simulink model "analyze"  (R2014a)
settings: Solver=FixedStepDiscrete  StartTime=0.0  StopTime=1  FixedStep=0.02  RelTol=1e-3
InitFcn:
  | Veh_Par_wxt
values from neighbouring files (symbols this model uses):
  ag_thr = 0.4*g    (= 3.924)    [Veh_Par_wxt.m]
  B = 2.25    [Veh_Par_wxt.m]
  bra_pre_em = 12    [Veh_Par_wxt.m]
  bra_pre_gz2 = 12/3    (= 4)    [Veh_Par_wxt.m]
  bra_pre_gz34 = 12/3    (= 4)    [Veh_Par_wxt.m]
  bra_pre_yd = 12/2    (= 6)    [Veh_Par_wxt.m]
  brakepre_dem_data = [0 1 2 3 4 5 6 7 8 9 10 11 12]    [Veh_Par_wxt.m]
  brakeTrq_dem_data = [0 218.198 436.396 654.594 872.792 1090.99 1309.188 1527.386 1745.584 1963.782 2181.98 2400.178 2618.376]    [Veh_Par_wxt.m]
  bratrq_max = 4*2618.376    (= 10473.504)    [Veh_Par_wxt.m]
  eff_tran = 0.75    [Veh_Par_wxt.m]
  G = Mass*g    (= 36297)    [Veh_Par_wxt.m]
  kd1 = 1    [Veh_Par_wxt.m]
  kd2 = 1    [Veh_Par_wxt.m]
  kd3 = 1    [Veh_Par_wxt.m]
  ki1 = 1    [Veh_Par_wxt.m]
  ki2 = 1    [Veh_Par_wxt.m]
  ki3 = 1    [Veh_Par_wxt.m]
  kp1 = 1    [Veh_Par_wxt.m]
  kp2 = 1    [Veh_Par_wxt.m]
  kp3 = 1    [Veh_Par_wxt.m]
  L = 3.12    [Veh_Par_wxt.m]
  premax = 12    [Veh_Par_wxt.m]
  Radius = 0.20    (= 0.2)    [Veh_Par_wxt.m]
  s_opt_yi_add = 0.05    [Veh_Par_wxt.m]
  s_opt_zhuan_add = 0.05    [Veh_Par_wxt.m]
  spd_map_mot = [0 100 200 300 360 400 500 600 700 800 900]*tras_ratio    [Veh_Par_wxt.m]
  spdmax = 900*tras_ratio    (= 5580)    [Veh_Par_wxt.m]
  speed_thr_park = 5/3.6/Radius*30/pi    (= 66.3145596216)    [Veh_Par_wxt.m]
  tras_ratio = 6.2    [Veh_Par_wxt.m]
  trq_map_mot = [1200 1200 1200 1200 1200 1080 864 720 617 540 480]/tras_ratio    [Veh_Par_wxt.m]
  trqmax = 80    [Veh_Par_wxt.m]
  v_thr1_b = 5    [Veh_Par_wxt.m]
  v_thr2_b = 20    [Veh_Par_wxt.m]
  v_thr_park = 5    [Veh_Par_wxt.m]
undefined symbols (not defined in the file or in its folder): DiscIntNeverNeededParam
libraries: simulink x231, ec5744lib x19
(part 14 of 16)

== system analyze/MainControl/mode_control/forward/forward/Drive/驱动防滑控制TCS/转向TCS/右转 ==
  trq_dem_lf : Inport
  trq_dem_lr : Inport  Port=2
  trq_dem_rf : Inport  Port=3
  trq_dem_rr : Inport  Port=4
  bra_pre_l : Inport  Port=5
  bra_pre_r : Inport  Port=6
  s_act_lf : Inport  Port=7
  s_act_lr : Inport  Port=8
  s_act_rf : Inport  Port=9
  s_act_rr : Inport  Port=10
  brake_dem : Inport  Port=11
  s_opt_zhuan : Inport  Port=12
  Action Port : ActionPort  ActionType=case
  Constant{,1..3} (4 alike) : Constant  Value=s_opt_zhuan_add
  Constant4 : Constant  Value=0
  Constant5 : Constant  Value=0
  MATLAB Function : MATLAB Function  TreatAsAtomicUnit=on
  MATLAB Function1 : MATLAB Function  TreatAsAtomicUnit=on
  MATLAB Function2 : MATLAB Function  TreatAsAtomicUnit=on
  MATLAB Function3 : MATLAB Function  TreatAsAtomicUnit=on
  MATLAB Function4 : MATLAB Function  TreatAsAtomicUnit=on
  Memory{,1..3} (4 alike) : Memory  InheritSampleTime=on
  Multiport Switch : MultiPortSwitch  DataPortOrder=Zero-based contiguous  Inputs=4
  Mux{,1..3} (4 alike) : Mux  Inputs=6
  Switch Case : SwitchCase  CaseConditions={0,1,2,3}  ShowDefaultCase=off
  Terminator{,1..3} (4 alike) : Terminator
  前后轮均滑转 : Subsystem  TreatAsAtomicUnit=on
  前轮滑转 : Subsystem  TreatAsAtomicUnit=on
  后轮滑转 : Subsystem  TreatAsAtomicUnit=on
  无滑转 : Subsystem  TreatAsAtomicUnit=on
  forward_dem : Outport
  wires:
  Mux3/1 -> Multiport Switch/5
  [s_opt_zhuan] -> 前后轮均滑转/10(s_opt_zhuan)
  [s_act_lr] -> 前后轮均滑转/9(s_act_lr)
  [s_act_lf] -> 前后轮均滑转/8(s_act_lf)
  Switch Case/4 -> 前后轮均滑转/Action
  前后轮均滑转/6(bra_pre_r1) -> Mux3/6
  前后轮均滑转/5(bra_pre_l1) -> Mux3/5
  前后轮均滑转/4(mot_rr) -> Mux3/4
  前后轮均滑转/2(mot_lr) -> Mux3/2
  前后轮均滑转/3(mot_rf) -> Mux3/3
  前后轮均滑转/1(mot_lf) -> Mux3/1
  Switch Case/3 -> 后轮滑转/Action
  [s_opt_zhuan] -> 后轮滑转/9(s_opt_zhuan)
  [s_act_lr] -> 后轮滑转/8(s_act_lr)
  Mux2/1 -> Multiport Switch/4
  后轮滑转/6(bra_pre_r1) -> Mux2/6
  后轮滑转/5(bra_pre_l1) -> Mux2/5
  后轮滑转/4(mot_rr) -> Mux2/4
  后轮滑转/2(mot_lr) -> Mux2/2
  后轮滑转/3(mot_rf) -> Mux2/3
  后轮滑转/1(mot_lf) -> Mux2/1
  [s_opt_zhuan] -> 前轮滑转/9(s_opt_zhuan)
  [s_act_lf] -> 前轮滑转/8(s_act_lf)
  Mux1/1 -> Multiport Switch/3
  前轮滑转/4(mot_rr) -> Mux1/4
  前轮滑转/5(bra_pre_l1) -> Mux1/5
  前轮滑转/1(mot_lf) -> Mux1/1
  前轮滑转/2(mot_lr) -> Mux1/2
  前轮滑转/3(mot_rf) -> Mux1/3
  前轮滑转/6(bra_pre_r1) -> Mux1/6
  Switch Case/2 -> 前轮滑转/Action
  Multiport Switch/1 -> forward_dem/1
  Mux/1 -> Multiport Switch/2
  无滑转/6(bra_pre_r1) -> Mux/6
  无滑转/5(bra_pre_l1) -> Mux/5
  无滑转/3(mot_rf) -> Mux/3
  无滑转/4(mot_rr) -> Mux/4
  无滑转/2(mot_lr) -> Mux/2
  无滑转/1(mot_lf) -> Mux/1
  brake_dem/1 -> 前轮滑转/7(brake_dem), 后轮滑转/7(brake_dem), 前后轮均滑转/7(brake_dem), 无滑转/7(brake_dem)
  bra_pre_r/1 -> 前轮滑转/6(bra_pre_r), 后轮滑转/6(bra_pre_r), 前后轮均滑转/6(bra_pre_r), 无滑转/6(bra_pre_r)
  bra_pre_l/1 -> 前轮滑转/5(bra_pre_l), 后轮滑转/5(bra_pre_l), 前后轮均滑转/5(bra_pre_l), 无滑转/5(bra_pre_l)
  trq_dem_rr/1 -> 前轮滑转/4(trq_dem_rr), 后轮滑转/4(trq_dem_rr), 前后轮均滑转/4(trq_dem_rr), 无滑转/4(trq_dem_rr)
  trq_dem_rf/1 -> 前轮滑转/3(trq_dem_rf), 后轮滑转/3(trq_dem_rf), 前后轮均滑转/3(trq_dem_rf), 无滑转/3(trq_dem_rf)
  trq_dem_lr/1 -> 后轮滑转/2(trq_dem_lr), 前后轮均滑转/2(trq_dem_lr), 前轮滑转/2(trq_dem_lr), 无滑转/2(trq_dem_lr)
  trq_dem_lf/1 -> 前轮滑转/1(trq_dem_lf), 后轮滑转/1(trq_dem_lf), 前后轮均滑转/1(trq_dem_lf), 无滑转/1(trq_dem_lf)
  Switch Case/1 -> 无滑转/Action
  MATLAB Function4/1(y) -> Switch Case/1, Multiport Switch/1
  [flag_lr] -> MATLAB Function4/2(flag_lr)
  [flag_lf] -> MATLAB Function4/1(flag_lf)
  Constant3/1 -> MATLAB Function3/3(s_opt_zhuan_add)
  Memory3/1 -> MATLAB Function3/4(flag_rr_pre)
  MATLAB Function3/1(flag_rr) -> Terminator1/1, Memory3/1
  s_opt_zhuan/1 -> MATLAB Function/2(s_opt_zhuan), MATLAB Function1/2(s_opt_zhuan), MATLAB Function2/2(s_opt_zhuan), MATLAB Function3/2(s_opt_zhuan), [s_opt_zhuan]
  s_act_rr/1 -> MATLAB Function3/1(s_act_rr)
  Constant2/1 -> MATLAB Function2/3(s_opt_zhuan_add)
  Memory2/1 -> MATLAB Function2/4(flag_rf_pre)
  MATLAB Function2/1(flag_rf) -> Terminator/1, Memory2/1
  s_act_rf/1 -> MATLAB Function2/1(s_act_rf)
  Constant1/1 -> MATLAB Function1/3(s_opt_zhuan_add)
  Memory1/1 -> MATLAB Function1/4(flag_lr_pre)
  MATLAB Function1/1(flag_lr) -> Terminator3/1, Memory1/1
  s_act_lr/1 -> [s_act_lr], MATLAB Function1/1(s_act_lr)
  Constant/1 -> MATLAB Function/3(s_opt_zhuan_add)
  Memory/1 -> MATLAB Function/4(flag_lf_pre)
  MATLAB Function/1(flag_lf) -> Terminator2/1, Memory/1
  s_act_lf/1 -> [s_act_lf], MATLAB Function/1(s_act_lf)
  Constant4/1 -> [flag_lf]
  Constant5/1 -> [flag_lr]

== system analyze/MainControl/mode_control/forward/forward/Drive/驱动防滑控制TCS/转向TCS/左转 ==
  trq_dem_lf : Inport
  trq_dem_lr : Inport  Port=2
  trq_dem_rf : Inport  Port=3
  trq_dem_rr : Inport  Port=4
  bra_pre_l : Inport  Port=5
  bra_pre_r : Inport  Port=6
  s_act_lf : Inport  Port=7
  s_act_lr : Inport  Port=8
  s_act_rf : Inport  Port=9
  s_act_rr : Inport  Port=10
  brake_dem : Inport  Port=11
  s_opt_zhuan : Inport  Port=12
  Action Port : ActionPort  ActionType=case
  Constant{,1..3} (4 alike) : Constant  Value=s_opt_zhuan_add
  Constant4 : Constant  Value=0
  Constant5 : Constant  Value=0
  MATLAB Function : MATLAB Function  TreatAsAtomicUnit=on
  MATLAB Function1 : MATLAB Function  TreatAsAtomicUnit=on
  MATLAB Function2 : MATLAB Function  TreatAsAtomicUnit=on
  MATLAB Function3 : MATLAB Function  TreatAsAtomicUnit=on
  MATLAB Function4 : MATLAB Function  TreatAsAtomicUnit=on
  Memory{,1..3} (4 alike) : Memory  InheritSampleTime=on
  Multiport Switch : MultiPortSwitch  DataPortOrder=Zero-based contiguous  Inputs=4
  Mux{,1..3} (4 alike) : Mux  Inputs=6
  Switch Case : SwitchCase  CaseConditions={0,1,2,3}  ShowDefaultCase=off
  Terminator{,1..3} (4 alike) : Terminator
  前后轮均滑转 : Subsystem  TreatAsAtomicUnit=on
  前轮滑转 : Subsystem  TreatAsAtomicUnit=on
  后轮滑转 : Subsystem  TreatAsAtomicUnit=on
  无滑转 : Subsystem  TreatAsAtomicUnit=on
  forward_dem : Outport
  wires:
  s_act_lf/1 -> MATLAB Function/1(s_act_lf)
  MATLAB Function/1(flag_lf) -> Terminator/1, Memory/1
  Memory/1 -> MATLAB Function/4(flag_lf_pre)
  Constant/1 -> MATLAB Function/3(s_opt_zhuan_add)
  s_act_lr/1 -> MATLAB Function1/1(s_act_lr)
  MATLAB Function1/1(flag_lr) -> Terminator1/1, Memory1/1
  Memory1/1 -> MATLAB Function1/4(flag_lr_pre)
  Constant1/1 -> MATLAB Function1/3(s_opt_zhuan_add)
  s_act_rf/1 -> [s_act_rf], MATLAB Function2/1(s_act_rf)
  MATLAB Function2/1(flag_rf) -> Terminator2/1, Memory2/1
  Memory2/1 -> MATLAB Function2/4(flag_rf_pre)
  Constant2/1 -> MATLAB Function2/3(s_opt_zhuan_add)
  s_act_rr/1 -> [s_act_rr], MATLAB Function3/1(s_act_rr)
  s_opt_zhuan/1 -> [s_opt_zhuan], MATLAB Function3/2(s_opt_zhuan), MATLAB Function2/2(s_opt_zhuan), MATLAB Function1/2(s_opt_zhuan), MATLAB Function/2(s_opt_zhuan)
  MATLAB Function3/1(flag_rr) -> Terminator3/1, Memory3/1
  Memory3/1 -> MATLAB Function3/4(flag_rr_pre)
  Constant3/1 -> MATLAB Function3/3(s_opt_zhuan_add)
  [flag_rf] -> MATLAB Function4/1(flag_rf)
  [flag_rr] -> MATLAB Function4/2(flag_rr)
  MATLAB Function4/1(y) -> Multiport Switch/1, Switch Case/1
  Switch Case/1 -> 无滑转/Action
  trq_dem_lf/1 -> 无滑转/1(trq_dem_lf), 前后轮均滑转/1(trq_dem_lf), 后轮滑转/1(trq_dem_lf), 前轮滑转/1(trq_dem_lf)
  trq_dem_lr/1 -> 无滑转/2(trq_dem_lr), 前轮滑转/2(trq_dem_lr), 前后轮均滑转/2(trq_dem_lr), 后轮滑转/2(trq_dem_lr)
  trq_dem_rf/1 -> 无滑转/3(trq_dem_rf), 前后轮均滑转/3(trq_dem_rf), 后轮滑转/3(trq_dem_rf), 前轮滑转/3(trq_dem_rf)
  trq_dem_rr/1 -> 无滑转/4(trq_dem_rr), 前后轮均滑转/4(trq_dem_rr), 后轮滑转/4(trq_dem_rr), 前轮滑转/4(trq_dem_rr)
  bra_pre_l/1 -> 无滑转/5(bra_pre_l), 前后轮均滑转/5(bra_pre_l), 后轮滑转/5(bra_pre_l), 前轮滑转/5(bra_pre_l)
  bra_pre_r/1 -> 无滑转/6(bra_pre_r), 前后轮均滑转/6(bra_pre_r), 后轮滑转/6(bra_pre_r), 前轮滑转/6(bra_pre_r)
  brake_dem/1 -> 无滑转/7(brake_dem), 前后轮均滑转/7(brake_dem), 后轮滑转/7(brake_dem), 前轮滑转/7(brake_dem)
  无滑转/1(mot_lf) -> Mux/1
  无滑转/2(mot_lr) -> Mux/2
  无滑转/4(mot_rr) -> Mux/4
  无滑转/3(mot_rf) -> Mux/3
  无滑转/5(bra_pre_l1) -> Mux/5
  无滑转/6(bra_pre_r1) -> Mux/6
  Mux/1 -> Multiport Switch/2
  Multiport Switch/1 -> forward_dem/1
  Switch Case/2 -> 前轮滑转/Action
  前轮滑转/6(bra_pre_r1) -> Mux1/6
  前轮滑转/3(mot_rf) -> Mux1/3
  前轮滑转/2(mot_lr) -> Mux1/2
  前轮滑转/1(mot_lf) -> Mux1/1
  前轮滑转/5(bra_pre_l1) -> Mux1/5
  前轮滑转/4(mot_rr) -> Mux1/4
  Mux1/1 -> Multiport Switch/3
  [s_act_rf] -> 前轮滑转/8(s_act_rf)
  [s_opt_zhuan] -> 前轮滑转/9(s_opt_zhuan)
  后轮滑转/1(mot_lf) -> Mux2/1
  后轮滑转/3(mot_rf) -> Mux2/3
  后轮滑转/2(mot_lr) -> Mux2/2
  后轮滑转/4(mot_rr) -> Mux2/4
  后轮滑转/5(bra_pre_l1) -> Mux2/5
  后轮滑转/6(bra_pre_r1) -> Mux2/6
  Mux2/1 -> Multiport Switch/4
  [s_act_rr] -> 后轮滑转/8(s_act_rr)
  [s_opt_zhuan] -> 后轮滑转/9(s_opt_zhuan)
  Switch Case/3 -> 后轮滑转/Action
  前后轮均滑转/1(mot_lf) -> Mux3/1
  前后轮均滑转/3(mot_rf) -> Mux3/3
  前后轮均滑转/2(mot_lr) -> Mux3/2
  前后轮均滑转/4(mot_rr) -> Mux3/4
  前后轮均滑转/5(bra_pre_l1) -> Mux3/5
  前后轮均滑转/6(bra_pre_r1) -> Mux3/6
  Switch Case/4 -> 前后轮均滑转/Action
  [s_act_rf] -> 前后轮均滑转/8(s_act_rf)
  [s_act_rr] -> 前后轮均滑转/9(s_act_rr)
  [s_opt_zhuan] -> 前后轮均滑转/10(s_opt_zhuan)
  Mux3/1 -> Multiport Switch/5
  Constant4/1 -> [flag_rf]
  Constant5/1 -> [flag_rr]

== matlab function analyze/MainControl/mode_control/backward/backward/Drive/驱动防滑控制TCS/直行TCS/直行/HeartBeat ==
  data: life_pre input; life output
function life = fcn(life_pre)
%#codegen
life=life_pre+1;
if life>15
    life=0;
end
end

== matlab function analyze/MainControl/mode_control/backward/backward/Drive/驱动防滑控制TCS/直行TCS/直行/MATLAB Function4 ==
  data: trq_dem_lf input; trq_dem_lr input; trq_dem_rf input; trq_dem_rr input; bra_pre_l input; bra_pre_r input; brakepre_dem input; flag_lf input; flag_lr input; trq_out_lf output; flag_rf input; flag_rr input; trq_out_lr output; trq_out_rf output; trq_out_rr output; trq_pid_lf input; trq_pid_lr input; trq_pid_rf input; trq_pid_rr input; brapre_out_l output; brapre_out_r output; mode output
function [trq_out_lf,trq_out_lr,trq_out_rf,trq_out_rr,brapre_out_l,brapre_out_r,mode] = fcn(trq_dem_lf,trq_dem_lr,trq_dem_rf,trq_dem_rr,bra_pre_l,bra_pre_r,brakepre_dem,flag_lf,flag_lr,flag_rf,flag_rr,trq_pid_lf,trq_pid_lr,trq_pid_rf,trq_pid_rr)
%#codegen pid模块在外面做，里面进行十六种情况的判断，先看一下效果，不能再修改。
if flag_lf==0 && flag_lr==0 && flag_rf==0 && flag_rr==0 % 0电机滑转===============================================0电机滑转
    trq_out_lf=trq_dem_lf;
    trq_out_lr=trq_dem_lr;
    trq_out_rf=trq_dem_rf;
    trq_out_rr=trq_dem_rr;
    brapre_out_l=bra_pre_l+brakepre_dem;
    brapre_out_r=bra_pre_r+brakepre_dem;
    mode=1;
elseif flag_lf==1 && flag_lr==0 &&flag_rf==0 && flag_rr==0 %左前轮滑转===================================================1电机滑转
    trq_out_lf=trq_pid_lf;
    trq_out_lr=trq_dem_lr+(trq_dem_lf-trq_out_lf);
    trq_out_rf=trq_dem_rf;
    trq_out_rr=trq_dem_rr;
    brapre_out_l=bra_pre_l+brakepre_dem;
    brapre_out_r=bra_pre_r+brakepre_dem;
    mode=2;
elseif flag_lf==0 && flag_lr==1 &&flag_rf==0 && flag_rr==0 %左后轮滑转
    trq_out_lr=trq_pid_lr;
    trq_out_lf=trq_dem_lf+(trq_dem_lr-trq_out_lr);
    trq_out_rf=trq_dem_rf;
    trq_out_rr=trq_dem_rr;
    brapre_out_l=bra_pre_l+brakepre_dem;
    brapre_out_r=bra_pre_r+brakepre_dem;
    mode=3;
elseif flag_lf==0 && flag_lr==0 &&flag_rf==1 && flag_rr==0 %右前轮滑转
    trq_out_rf=trq_pid_rf;
    trq_out_rr=trq_dem_rr+(trq_dem_rf-trq_out_rf);
    trq_out_lf=trq_dem_lf;
    trq_out_lr=trq_dem_lr;
    brapre_out_l=bra_pre_l+brakepre_dem;
    brapre_out_r=bra_pre_r+brakepre_dem;
    mode=4;
elseif flag_lf==0 && flag_lr==0 &&flag_rf==0 && flag_rr==1 %右后轮滑转
    trq_out_rr=trq_pid_rr;
    trq_out_rf=trq_dem_rf+(trq_dem_rr-trq_out_rr);
    trq_out_lf=trq_dem_lf;
    trq_out_lr=trq_dem_lr;
    brapre_out_l=bra_pre_l+brakepre_dem;
    brapre_out_r=bra_pre_r+brakepre_dem;
    mode=5;
elseif flag_lf==1 && flag_lr==1 &&flag_rf==0 && flag_rr==0 %左侧两轮滑转=====================================================================2电机滑转
    trq_out_lf=trq_pid_lf;
    trq_out_lr=trq_pid_lr;
    trq_out_rf=trq_dem_rf-(trq_dem_lf+trq_dem_lr-trq_out_lf-trq_out_lr)/2;
    trq_out_rr=trq_dem_rr-(trq_dem_lf+trq_dem_lr-trq_out_lf-trq_out_lr)/2;
    brapre_out_l=bra_pre_l+brakepre_dem;
    brapre_out_r=bra_pre_r+brakepre_dem;
    mode=6;
elseif flag_lf==0 && flag_lr==0 &&flag_rf==1 && flag_rr==1 %右侧两轮滑转
    trq_out_rf=trq_pid_rf;
    trq_out_rr=trq_pid_rr;
    trq_out_lf=trq_dem_lf-(trq_dem_rf+trq_dem_rr-trq_out_rf-trq_out_rr)/2;
    trq_out_lr=trq_dem_lr-(trq_dem_rf+trq_dem_rr-trq_out_rf-trq_out_rr)/2;
    brapre_out_l=bra_pre_l+brakepre_dem;
    brapre_out_r=bra_pre_r+brakepre_dem;
    mode=7;
elseif flag_lf==1 && flag_lr==0 &&flag_rf==1 && flag_rr==0 %前轴滑转
    trq_out_lf=trq_pid_lf;
    trq_out_lr=trq_dem_lr+(trq_dem_lf-trq_out_lf);
    trq_out_rf=trq_pid_rf;
    trq_out_rr=trq_dem_rr+(trq_dem_rf-trq_out_rf);
    brapre_out_l=bra_pre_l+brakepre_dem;
    brapre_out_r=bra_pre_r+brakepre_dem;
    mode=8;
elseif flag_lf==0 && flag_lr==1 &&flag_rf==0 && flag_rr==1 %后轴滑转
    trq_out_lr=trq_pid_lr;
    trq_out_lf=trq_dem_lf+(trq_dem_lr-trq_out_lr);
    trq_out_rr=trq_pid_rr;
    trq_out_rf=trq_dem_rf+(trq_dem_rr-trq_out_rr);
    brapre_out_l=bra_pre_l+brakepre_dem;
    brapre_out_r=bra_pre_r+brakepre_dem;
    mode=9;
elseif flag_lf==1 && flag_lr==0 &&flag_rf==0 && flag_rr==1 %左前轮和右后轮滑转
    trq_out_lf=trq_pid_lf;
    trq_out_lr=trq_dem_lr+(trq_dem_lf-trq_out_lf);
    trq_out_rr=trq_pid_rr;
    trq_out_rf=trq_dem_rf+(trq_dem_rr-trq_out_rr);
    brapre_out_l=bra_pre_l+brakepre_dem;
    brapre_out_r=bra_pre_r+brakepre_dem;
    mode=10;
elseif flag_lf==0 && flag_lr==1 &&flag_rf==1 && flag_rr==0 %左后轮和右前轮滑转
    trq_out_lr=trq_pid_lr;
    trq_out_lf=trq_dem_lf+(trq_dem_lr-trq_out_lr);
    trq_out_rf=trq_pid_rf;
    trq_out_rr=trq_dem_rr+(trq_dem_rf-trq_out_rf);
    brapre_out_l=bra_pre_l+brakepre_dem;
    brapre_out_r=bra_pre_r+brakepre_dem;
    mode=11;
elseif flag_lf==1 && flag_lr==1 &&flag_rf==1 && flag_rr==0 %右后不滑转======================================================================3电机滑转
    trq_out_lf=trq_pid_lf;
    trq_out_lr=trq_pid_lr;
    trq_out_rf=trq_pid_rf;
    trq_out_rr=trq_dem_rr+(trq_dem_rf-trq_out_rf)-(trq_dem_lf+trq_dem_lr-trq_out_lf-trq_out_lr);
    brapre_out_l=bra_pre_l+brakepre_dem;
    brapre_out_r=bra_pre_r+brakepre_dem;
    mode=12;
elseif flag_lf==1 && flag_lr==1 &&flag_rf==0 && flag_rr==1 %右前不滑转
    trq_out_lf=trq_pid_lf;
    trq_out_lr=trq_pid_lr;
    trq_out_rr=trq_pid_rr;
    trq_out_rf=trq_dem_rf+(trq_dem_rr-trq_out_rr)-(trq_dem_lf+trq_dem_lr-trq_out_lf-trq_out_lr);
    brapre_out_l=bra_pre_l+brakepre_dem;
    brapre_out_r=bra_pre_r+brakepre_dem;
    mode=13;
elseif flag_lf==1 && flag_lr==0 &&flag_rf==1 && flag_rr==1 %左后不滑转
    trq_out_rf=trq_pid_rf;
    trq_out_rr=trq_pid_rr;
    trq_out_lf=trq_pid_lf;
    trq_out_lr=trq_dem_lr+(trq_dem_lf-trq_out_lf)-(trq_dem_rf+trq_dem_rr-trq_out_rf-trq_out_rr);
    brapre_out_l=bra_pre_l+brakepre_dem;
    brapre_out_r=bra_pre_r+brakepre_dem;
    mode=14;
elseif flag_lf==0 && flag_lr==1 &&flag_rf==1 && flag_rr==1 %左前不滑转
    trq_out_rf=trq_pid_rf;
    trq_out_rr=trq_pid_rr;
    trq_out_lr=trq_pid_lr;
    trq_out_lf=trq_dem_lf+(trq_dem_lr-trq_out_lr)-(trq_dem_rf+trq_dem_rr-trq_out_rf-trq_out_rr);
    brapre_out_l=bra_pre_l+brakepre_dem;
    brapre_out_r=bra_pre_r+brakepre_dem;
    mode=15;
else
    %     flag_lf==1 && flag_lr==1 &&flag_rf==1 && flag_rr==1 %4电机均滑转======================================================================4电机均滑转
    trqcha=(trq_pid_lf+trq_pid_lr)-(trq_pid_rf+trq_pid_rr);
    if trqcha>0
        trq_out_rf=trq_pid_rf;
        trq_out_rr=trq_pid_rr;
        trq_out_lf=trq_pid_lf-(trq_pid_lf/(trq_pid_lf+trq_pid_lr))*trqcha;
        trq_out_lr=trq_pid_lr-(trq_pid_lr/(trq_pid_lf+trq_pid_lr))*trqcha;
    else
        trq_out_lf=trq_pid_lf;
        trq_out_lr=trq_pid_lr;
        trq_out_rf=trq_pid_rf+(trq_pid_rf/(trq_pid_rf+trq_pid_rr))*trqcha;
        trq_out_rr=trq_pid_rr+(trq_pid_rr/(trq_pid_rf+trq_pid_rr))*trqcha;
    end
    brapre_out_l=bra_pre_l+brakepre_dem;
    brapre_out_r=bra_pre_r+brakepre_dem;
    mode=16;
end
trq_out_lf=max(0,trq_out_lf);
trq_out_lr=max(0,trq_out_lr);
trq_out_rf=max(0,trq_out_rf);
trq_out_rr=max(0,trq_out_rr);
brapre_out_l=brapre_out_l;
brapre_out_r=brapre_out_r;
end

== system analyze/MainControl/mode_control/backward/backward/Drive/驱动防滑控制TCS/直行TCS/直行/Subsystem ==
  s_opt_zhuan : Inport
  s_act_lf : Inport  Port=2
  s_act_lr : Inport  Port=3
  s_act_rf : Inport  Port=4
  s_act_rr : Inport  Port=5
  flag_lf : Inport  Port=6
  flag_lr : Inport  Port=7
  flag_rf : Inport  Port=8
  flag_rr : Inport  Port=9
  trq_dem_lf : Inport  Port=10
  trq_dem_lr : Inport  Port=11
  trq_dem_rf : Inport  Port=12
  trq_dem_rr : Inport  Port=13
  Add{1..2,5,7} (4 alike) : Sum  Inputs=+++
  Add{3..4,6,8} (4 alike) : Sum
  Difference{,1..3} (4 alike) : simulink/Discrete/Difference  ICPrevInput=0.0  InputProcessing=Inherited  OutMin=[]  OutMax=[]  OutDataType=fixdt(1, 16)  OutScaling=2^-10  DoSatur=off
  Discrete-Time Integrator{,1..3} (4 alike) : DiscreteIntegrator  SampleTime=-1  ICPrevOutput=DiscIntNeverNeededParam  ICPrevScaledInput=DiscIntNeverNeededParam
  Gain{1,4,7,10} (4 alike) : Gain  Gain=kp2
  Gain{2,5,8,11} (4 alike) : Gain  Gain=ki2
  Gain{3,6,9,12} (4 alike) : Gain  Gain=kd2
  Gain{13..16} (4 alike) : Gain  Gain=1/tras_ratio
  Sum{,1..3} (4 alike) : Sum  Inputs=|+-
  Switch{,1..3} (4 alike) : Switch  Criteria=u2 > Threshold  Threshold=0.5
  trq_pid_lf : Outport
  trq_pid_lr : Outport  Port=2
  trq_pid_rf : Outport  Port=3
  trq_pid_rr : Outport  Port=4
  wires:
  Difference2/1 -> Add5/3
  Discrete-Time Integrator2/1 -> Add5/2
  Difference3/1 -> Add7/3
  Discrete-Time Integrator3/1 -> Add7/2
  Difference1/1 -> Add1/3
  Discrete-Time Integrator1/1 -> Add1/2
  Difference/1 -> Add2/3
  Discrete-Time Integrator/1 -> Add2/2
  Add5/1 -> Gain16/1
  Sum2/1 -> Gain7/1, Gain9/1, Gain8/1
  Sum3/1 -> Gain10/1, Gain12/1, Gain11/1
  Add7/1 -> Gain15/1
  Gain6/1 -> Difference1/1
  Add1/1 -> Gain14/1
  Sum1/1 -> Gain4/1, Gain6/1, Gain5/1
  Sum/1 -> Gain1/1, Gain3/1, Gain2/1
  Add2/1 -> Gain13/1
  Switch3/1 -> trq_pid_rf/1
  flag_rf/1 -> Switch3/2
  [s_opt_zhuan] -> Sum3/1
  Gain10/1 -> Add7/1
  Gain11/1 -> Discrete-Time Integrator3/1
  Gain12/1 -> Difference3/1
  s_act_rf/1 -> Sum3/2
  trq_dem_rf/1 -> Add8/2, Switch3/3
  Add8/1 -> Switch3/1
  Switch2/1 -> trq_pid_rr/1
  flag_rr/1 -> Switch2/2
  [s_opt_zhuan] -> Sum2/1
  Gain7/1 -> Add5/1
  Gain8/1 -> Discrete-Time Integrator2/1
  Gain9/1 -> Difference2/1
  s_act_rr/1 -> Sum2/2
  trq_dem_rr/1 -> Add6/2, Switch2/3
  Add6/1 -> Switch2/1
  Switch1/1 -> trq_pid_lr/1
  flag_lr/1 -> Switch1/2
  [s_opt_zhuan] -> Sum1/1
  Gain4/1 -> Add1/1
  Gain5/1 -> Discrete-Time Integrator1/1
  s_act_lr/1 -> Sum1/2
  trq_dem_lr/1 -> Add4/2, Switch1/3
  Add4/1 -> Switch1/1
  Switch/1 -> trq_pid_lf/1
  flag_lf/1 -> Switch/2
  s_opt_zhuan/1 -> Sum/1, [s_opt_zhuan]
  Gain1/1 -> Add2/1
  Gain2/1 -> Discrete-Time Integrator/1
  Gain3/1 -> Difference/1
  s_act_lf/1 -> Sum/2
  trq_dem_lf/1 -> Add3/2, Switch/3
  Add3/1 -> Switch/1
  Gain13/1 -> Add3/1
  Gain14/1 -> Add4/1
  Gain15/1 -> Add8/1
  Gain16/1 -> Add6/1

== system analyze/MainControl/mode_control/backward/backward/Drive/驱动防滑控制TCS/直行TCS/直行/Subsystem1 ==
  brake_dem : Inport
  1-D Lookup Table : Lookup_n-D  NumberOfTableDimensions=1  BreakpointsForDimension1=brakeTrq_dem_data  Table=brakepre_dem_data  InternalRulePriority=Speed  RndMeth=Simplest  InputSameDT=on
  Constant : Constant  Value=bratrq_max
  Gain1 : Gain  Gain=1/2
  Gain2 : Gain  Gain=1/100
  Gain3 : Gain  Gain=1/2
  Product : Product
  brakepre_dem : Outport
  wires:
  brake_dem/1 -> Gain2/1
  Gain3/1 -> 1-D Lookup Table/1
  Gain2/1 -> Product/2
  Gain1/1 -> Gain3/1
  Product/1 -> Gain1/1
  Constant/1 -> Product/1
  1-D Lookup Table/1 -> brakepre_dem/1

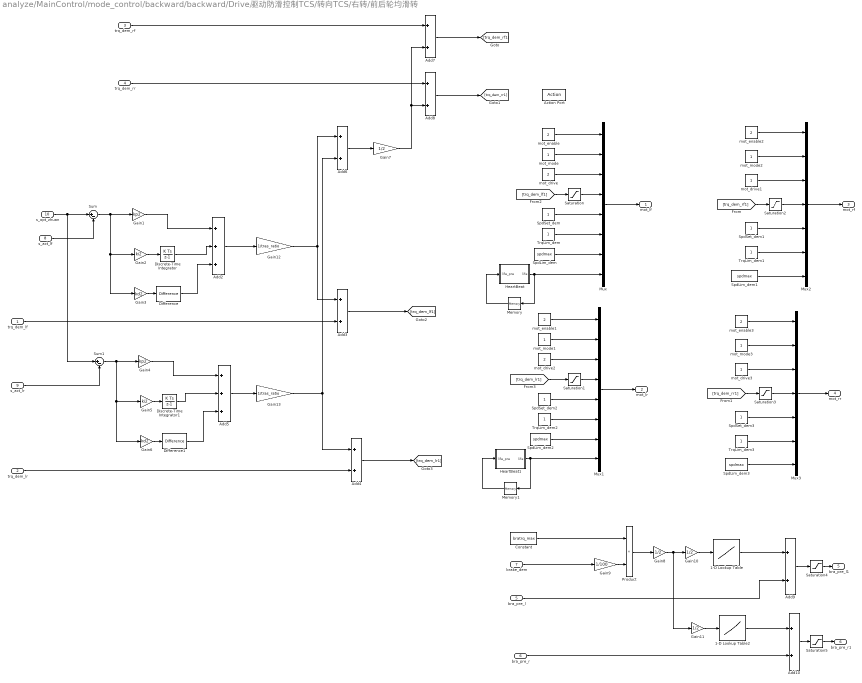
== system analyze/MainControl/mode_control/backward/backward/Drive/驱动防滑控制TCS/转向TCS/右转/前后轮均滑转 ==
  trq_dem_lf : Inport
  trq_dem_lr : Inport  Port=2
  trq_dem_rf : Inport  Port=3
  trq_dem_rr : Inport  Port=4
  bra_pre_l : Inport  Port=5
  bra_pre_r : Inport  Port=6
  brake_dem : Inport  Port=7
  s_act_lf : Inport  Port=8
  s_act_lr : Inport  Port=9
  s_opt_zhuan : Inport  Port=10
  Action Port : ActionPort  ActionType=case
  1-D Lookup Table : Lookup_n-D  NumberOfTableDimensions=1  BreakpointsForDimension1=brakeTrq_dem_data  Table=brakepre_dem_data  InternalRulePriority=Speed  RndMeth=Simplest  InputSameDT=on
  1-D Lookup Table2 : Lookup_n-D  NumberOfTableDimensions=1  BreakpointsForDimension1=brakeTrq_dem_data  Table=brakepre_dem_data  InternalRulePriority=Speed  RndMeth=Simplest  InputSameDT=on
  Add{3..4,6..10} (7 alike) : Sum
  Add2 : Sum  Inputs=+++
  Add5 : Sum  Inputs=+++
  Constant : Constant  Value=bratrq_max
  Difference : simulink/Discrete/Difference  ICPrevInput=0.0  InputProcessing=Inherited  OutMin=[]  OutMax=[]  OutDataType=fixdt(1, 16)  OutScaling=2^-10  DoSatur=off
  Difference1 : simulink/Discrete/Difference  ICPrevInput=0.0  InputProcessing=Inherited  OutMin=[]  OutMax=[]  OutDataType=fixdt(1, 16)  OutScaling=2^-10  DoSatur=off
  Discrete-Time Integrator : DiscreteIntegrator  SampleTime=-1  ICPrevOutput=DiscIntNeverNeededParam  ICPrevScaledInput=DiscIntNeverNeededParam
  Discrete-Time Integrator1 : DiscreteIntegrator  SampleTime=-1  ICPrevOutput=DiscIntNeverNeededParam  ICPrevScaledInput=DiscIntNeverNeededParam
  Gain1 : Gain  Gain=kp2
  Gain{7..8,10..11} (4 alike) : Gain  Gain=1/2
  Gain12 : Gain  Gain=1/tras_ratio
  Gain13 : Gain  Gain=1/tras_ratio
  Gain2 : Gain  Gain=ki2
  Gain3 : Gain  Gain=kd2
  Gain4 : Gain  Gain=kp2
  Gain5 : Gain  Gain=ki2
  Gain6 : Gain  Gain=kd2
  Gain9 : Gain  Gain=1/100
  HeartBeat : MATLAB Function  TreatAsAtomicUnit=on
  HeartBeat1 : MATLAB Function  TreatAsAtomicUnit=on
  Memory : Memory  InheritSampleTime=on
  Memory1 : Memory  InheritSampleTime=on
  Mux : Mux  Inputs=8
  Mux1 : Mux  Inputs=8
  Mux2 : Mux  Inputs=7
  Mux3 : Mux  Inputs=7
  Product : Product
  Saturation{,1..3} (4 alike) : Saturate  UpperLimit=trqmax  LowerLimit=-trqmax
  Saturation4 : Saturate  UpperLimit=premax  LowerLimit=0
  Saturation5 : Saturate  UpperLimit=premax  LowerLimit=0
  SpdLim_dem{,1..3} (4 alike) : Constant  Value=spdmax
  SpdSet_dem{,1..3} (4 alike) : Constant
  Sum : Sum  Inputs=|+-
  Sum1 : Sum  Inputs=|+-
  TrqLim_dem{,1..3} (4 alike) : Constant
  mot_drive : Constant  Value=2
  mot_drive1 : Constant
  mot_drive2 : Constant  Value=2
  mot_drive3 : Constant
  mot_enable{,1..3} (4 alike) : Constant  Value=2
  mot_mode{,1..3} (4 alike) : Constant
  mot_lf : Outport
  mot_lr : Outport  Port=2
  mot_rf : Outport  Port=3
  mot_rr : Outport  Port=4
  bra_pre_l1 : Outport  Port=5
  bra_pre_r1 : Outport  Port=6
  wires:
  Saturation5/1 -> bra_pre_r1/1
  Saturation4/1 -> bra_pre_l1/1
  Saturation3/1 -> Mux3/4
  Saturation2/1 -> Mux2/4
  Saturation1/1 -> Mux1/4
  Saturation/1 -> Mux/4
  Difference1/1 -> Add5/3
  Discrete-Time Integrator1/1 -> Add5/2
  Difference/1 -> Add2/3
  Discrete-Time Integrator/1 -> Add2/2
  Gain3/1 -> Difference/1
  brake_dem/1 -> Gain9/1
  Add10/1 -> Saturation5/1
  bra_pre_r/1 -> Add10/2
  1-D Lookup Table2/1 -> Add10/1
  Gain11/1 -> 1-D Lookup Table2/1
  Gain10/1 -> 1-D Lookup Table/1
  Gain9/1 -> Product/2
  Gain8/1 -> Gain10/1, Gain11/1
  Product/1 -> Gain8/1
  Constant/1 -> Product/1
  1-D Lookup Table/1 -> Add9/1
  Add9/1 -> Saturation4/1
  bra_pre_l/1 -> Add9/2
  SpdLim_dem3/1 -> Mux3/7
  TrqLim_dem3/1 -> Mux3/6
  Mux3/1 -> mot_rr/1
  SpdSet_dem3/1 -> Mux3/5
  mot_enable3/1 -> Mux3/1
  [trq_dem_rr1] -> Saturation3/1
  mot_mode3/1 -> Mux3/2
  mot_drive3/1 -> Mux3/3
  SpdLim_dem2/1 -> Mux1/7
  Memory1/1 -> HeartBeat1/1(life_pre)
  HeartBeat1/1(life) -> Memory1/1, Mux1/8
  TrqLim_dem2/1 -> Mux1/6
  Mux1/1 -> mot_lr/1
  SpdSet_dem2/1 -> Mux1/5
  mot_enable1/1 -> Mux1/1
  [trq_dem_lr1] -> Saturation1/1
  mot_mode1/1 -> Mux1/2
  mot_drive2/1 -> Mux1/3
  SpdLim_dem1/1 -> Mux2/7
  TrqLim_dem1/1 -> Mux2/6
  Mux2/1 -> mot_rf/1
  SpdSet_dem1/1 -> Mux2/5
  mot_enable2/1 -> Mux2/1
  [trq_dem_rf1] -> Saturation2/1
  mot_mode2/1 -> Mux2/2
  mot_drive1/1 -> Mux2/3
  SpdLim_dem/1 -> Mux/7
  Memory/1 -> HeartBeat/1(life_pre)
  HeartBeat/1(life) -> Memory/1, Mux/8
  TrqLim_dem/1 -> Mux/6
  Mux/1 -> mot_lf/1
  SpdSet_dem/1 -> Mux/5
  mot_enable/1 -> Mux/1
  [trq_dem_lf1] -> Saturation/1
  mot_mode/1 -> Mux/2
  mot_drive/1 -> Mux/3
  s_opt_zhuan/1 -> Sum1/1, Sum/1
  Sum/1 -> Gain2/1, Gain3/1, Gain1/1
  Gain1/1 -> Add2/1
  Gain2/1 -> Discrete-Time Integrator/1
  s_act_lf/1 -> Sum/2
  Add2/1 -> Gain12/1
  trq_dem_lf/1 -> Add3/2
  Add3/1 -> [trq_dem_lf1]
  Add4/1 -> [trq_dem_lr1]
  Sum1/1 -> Gain5/1, Gain6/1, Gain4/1
  Gain4/1 -> Add5/1
  Gain5/1 -> Discrete-Time Integrator1/1
  Gain6/1 -> Difference1/1
  s_act_lr/1 -> Sum1/2
  Add5/1 -> Gain13/1
  trq_dem_lr/1 -> Add4/2
  Add6/1 -> Gain7/1
  trq_dem_rf/1 -> Add7/1
  Gain7/1 -> Add8/2, Add7/2
  Add7/1 -> [trq_dem_rf1]
  trq_dem_rr/1 -> Add8/1
  Add8/1 -> [trq_dem_rr1]
  Gain12/1 -> Add3/1, Add6/1
  Gain13/1 -> Add4/1, Add6/2

== system analyze/MainControl/mode_control/backward/backward/Drive/驱动防滑控制TCS/转向TCS/右转/前轮滑转 ==
  trq_dem_lf : Inport
  trq_dem_lr : Inport  Port=2
  trq_dem_rf : Inport  Port=3
  trq_dem_rr : Inport  Port=4
  bra_pre_l : Inport  Port=5
  bra_pre_r : Inport  Port=6
  brake_dem : Inport  Port=7
  s_act_lf : Inport  Port=8
  s_opt_zhuan : Inport  Port=9
  Action Port : ActionPort  ActionType=case
  1-D Lookup Table : Lookup_n-D  NumberOfTableDimensions=1  BreakpointsForDimension1=brakeTrq_dem_data  Table=brakepre_dem_data  InternalRulePriority=Speed  RndMeth=Simplest  InputSameDT=on
  1-D Lookup Table2 : Lookup_n-D  NumberOfTableDimensions=1  BreakpointsForDimension1=brakeTrq_dem_data  Table=brakepre_dem_data  InternalRulePriority=Speed  RndMeth=Simplest  InputSameDT=on
  Add2 : Sum  Inputs=+++
  Add{3..6} (4 alike) : Sum
  Constant : Constant  Value=bratrq_max
  Difference : simulink/Discrete/Difference  ICPrevInput=0.0  InputProcessing=Inherited  OutMin=[]  OutMax=[]  OutDataType=fixdt(1, 16)  OutScaling=2^-10  DoSatur=off
  Discrete-Time Integrator : DiscreteIntegrator  SampleTime=-1  ICPrevOutput=DiscIntNeverNeededParam  ICPrevScaledInput=DiscIntNeverNeededParam
  Gain1 : Gain  Gain=kp2
  Gain2 : Gain  Gain=ki2
  Gain3 : Gain  Gain=kd2
  Gain4 : Gain  Gain=-1
  Gain5 : Gain  Gain=1/2
  Gain6 : Gain  Gain=1/100
  Gain7 : Gain  Gain=1/2
  Gain8 : Gain  Gain=1/2
  Gain9 : Gain  Gain=1/tras_ratio
  HeartBeat : MATLAB Function  TreatAsAtomicUnit=on
  HeartBeat1 : MATLAB Function  TreatAsAtomicUnit=on
  Memory : Memory  InheritSampleTime=on
  Memory1 : Memory  InheritSampleTime=on
  Mux : Mux  Inputs=8
  Mux1 : Mux  Inputs=8
  Mux2 : Mux  Inputs=7
  Mux3 : Mux  Inputs=7
  Product : Product
  Saturation{,1..3} (4 alike) : Saturate  UpperLimit=trqmax  LowerLimit=-trqmax
  Saturation4 : Saturate  UpperLimit=premax  LowerLimit=0
  Saturation5 : Saturate  UpperLimit=premax  LowerLimit=0
  SpdLim_dem{,1..3} (4 alike) : Constant  Value=spdmax
  SpdSet_dem{,1..3} (4 alike) : Constant
  Sum : Sum  Inputs=|+-
  TrqLim_dem{,1..3} (4 alike) : Constant
  mot_drive : Constant  Value=2
  mot_drive1 : Constant
  mot_drive2 : Constant  Value=2
  mot_drive3 : Constant
  mot_enable{,1..3} (4 alike) : Constant  Value=2
  mot_mode{,1..3} (4 alike) : Constant
  mot_lf : Outport
  mot_lr : Outport  Port=2
  mot_rf : Outport  Port=3
  mot_rr : Outport  Port=4
  bra_pre_l1 : Outport  Port=5
  bra_pre_r1 : Outport  Port=6
  wires:
  Saturation5/1 -> bra_pre_r1/1
  Saturation4/1 -> bra_pre_l1/1
  Saturation3/1 -> Mux3/4
  Saturation2/1 -> Mux2/4
  Saturation1/1 -> Mux1/4
  Saturation/1 -> Mux/4
  Difference/1 -> Add2/3
  Discrete-Time Integrator/1 -> Add2/2
  brake_dem/1 -> Gain6/1
  Add6/1 -> Saturation5/1
  bra_pre_r/1 -> Add6/2
  1-D Lookup Table2/1 -> Add6/1
  Gain8/1 -> 1-D Lookup Table2/1
  Gain7/1 -> 1-D Lookup Table/1
  Gain6/1 -> Product/2
  Gain5/1 -> Gain7/1, Gain8/1
  Product/1 -> Gain5/1
  Constant/1 -> Product/1
  1-D Lookup Table/1 -> Add5/1
  Add5/1 -> Saturation4/1
  bra_pre_l/1 -> Add5/2
  SpdLim_dem3/1 -> Mux3/7
  TrqLim_dem3/1 -> Mux3/6
  Mux3/1 -> mot_rr/1
  SpdSet_dem3/1 -> Mux3/5
  mot_enable3/1 -> Mux3/1
  trq_dem_rr/1 -> Saturation3/1
  mot_mode3/1 -> Mux3/2
  mot_drive3/1 -> Mux3/3
  SpdLim_dem2/1 -> Mux1/7
  Memory1/1 -> HeartBeat1/1(life_pre)
  HeartBeat1/1(life) -> Memory1/1, Mux1/8
  TrqLim_dem2/1 -> Mux1/6
  Mux1/1 -> mot_lr/1
  SpdSet_dem2/1 -> Mux1/5
  mot_enable1/1 -> Mux1/1
  [trq_dem_lr1] -> Saturation1/1
  mot_mode1/1 -> Mux1/2
  mot_drive2/1 -> Mux1/3
  SpdLim_dem1/1 -> Mux2/7
  TrqLim_dem1/1 -> Mux2/6
  Mux2/1 -> mot_rf/1
  SpdSet_dem1/1 -> Mux2/5
  mot_enable2/1 -> Mux2/1
  trq_dem_rf/1 -> Saturation2/1
  mot_mode2/1 -> Mux2/2
  mot_drive1/1 -> Mux2/3
  SpdLim_dem/1 -> Mux/7
  Memory/1 -> HeartBeat/1(life_pre)
  HeartBeat/1(life) -> Memory/1, Mux/8
  TrqLim_dem/1 -> Mux/6
  Mux/1 -> mot_lf/1
  SpdSet_dem/1 -> Mux/5
  mot_enable/1 -> Mux/1
  [trq_dem_lf1] -> Saturation/1
  mot_mode/1 -> Mux/2
  mot_drive/1 -> Mux/3
  s_opt_zhuan/1 -> Sum/1
  Sum/1 -> Gain2/1, Gain3/1, Gain1/1
  Gain1/1 -> Add2/1
  Gain2/1 -> Discrete-Time Integrator/1
  Gain3/1 -> Difference/1
  s_act_lf/1 -> Sum/2
  Add2/1 -> Gain9/1
  trq_dem_lf/1 -> Add3/2
  Add3/1 -> [trq_dem_lf1]
  Gain4/1 -> Add4/1
  trq_dem_lr/1 -> Add4/2
  Add4/1 -> [trq_dem_lr1]
  Gain9/1 -> Gain4/1, Add3/1

== system analyze/MainControl/mode_control/backward/backward/Drive/驱动防滑控制TCS/转向TCS/右转/后轮滑转 ==
  trq_dem_lf : Inport
  trq_dem_lr : Inport  Port=2
  trq_dem_rf : Inport  Port=3
  trq_dem_rr : Inport  Port=4
  bra_pre_l : Inport  Port=5
  bra_pre_r : Inport  Port=6
  brake_dem : Inport  Port=7
  s_act_lr : Inport  Port=8
  s_opt_zhuan : Inport  Port=9
  Action Port : ActionPort  ActionType=case
  1-D Lookup Table : Lookup_n-D  NumberOfTableDimensions=1  BreakpointsForDimension1=brakeTrq_dem_data  Table=brakepre_dem_data  InternalRulePriority=Speed  RndMeth=Simplest  InputSameDT=on
  1-D Lookup Table2 : Lookup_n-D  NumberOfTableDimensions=1  BreakpointsForDimension1=brakeTrq_dem_data  Table=brakepre_dem_data  InternalRulePriority=Speed  RndMeth=Simplest  InputSameDT=on
  Add2 : Sum  Inputs=+++
  Add{3..6} (4 alike) : Sum
  Constant : Constant  Value=bratrq_max
  Difference : simulink/Discrete/Difference  ICPrevInput=0.0  InputProcessing=Inherited  OutMin=[]  OutMax=[]  OutDataType=fixdt(1, 16)  OutScaling=2^-10  DoSatur=off
  Discrete-Time Integrator : DiscreteIntegrator  SampleTime=-1  ICPrevOutput=DiscIntNeverNeededParam  ICPrevScaledInput=DiscIntNeverNeededParam
  Gain1 : Gain  Gain=kp2
  Gain2 : Gain  Gain=ki2
  Gain3 : Gain  Gain=kd2
  Gain4 : Gain  Gain=-1
  Gain5 : Gain  Gain=1/2
  Gain6 : Gain  Gain=1/100
  Gain7 : Gain  Gain=1/2
  Gain8 : Gain  Gain=1/2
  Gain9 : Gain  Gain=1/tras_ratio
  HeartBeat : MATLAB Function  TreatAsAtomicUnit=on
  HeartBeat1 : MATLAB Function  TreatAsAtomicUnit=on
  Memory : Memory  InheritSampleTime=on
  Memory1 : Memory  InheritSampleTime=on
  Mux : Mux  Inputs=8
  Mux1 : Mux  Inputs=8
  Mux2 : Mux  Inputs=7
  Mux3 : Mux  Inputs=7
  Product : Product
  Saturation{,1..3} (4 alike) : Saturate  UpperLimit=trqmax  LowerLimit=-trqmax
  Saturation4 : Saturate  UpperLimit=premax  LowerLimit=0
  Saturation5 : Saturate  UpperLimit=premax  LowerLimit=0
  SpdLim_dem{,1..3} (4 alike) : Constant  Value=spdmax
  SpdSet_dem{,1..3} (4 alike) : Constant
  Sum : Sum  Inputs=|+-
  TrqLim_dem{,1..3} (4 alike) : Constant
  mot_drive : Constant  Value=2
  mot_drive1 : Constant
  mot_drive2 : Constant  Value=2
  mot_drive3 : Constant
  mot_enable{,1..3} (4 alike) : Constant  Value=2
  mot_mode{,1..3} (4 alike) : Constant
  mot_lf : Outport
  mot_lr : Outport  Port=2
  mot_rf : Outport  Port=3
  mot_rr : Outport  Port=4
  bra_pre_l1 : Outport  Port=5
  bra_pre_r1 : Outport  Port=6
  wires:
  Saturation5/1 -> bra_pre_r1/1
  Saturation4/1 -> bra_pre_l1/1
  Saturation3/1 -> Mux3/4
  Saturation2/1 -> Mux2/4
  Saturation1/1 -> Mux1/4
  Saturation/1 -> Mux/4
  Difference/1 -> Add2/3
  Discrete-Time Integrator/1 -> Add2/2
  brake_dem/1 -> Gain6/1
  Add6/1 -> Saturation5/1
  bra_pre_r/1 -> Add6/2
  1-D Lookup Table2/1 -> Add6/1
  Gain8/1 -> 1-D Lookup Table2/1
  Gain7/1 -> 1-D Lookup Table/1
  Gain6/1 -> Product/2
  Gain5/1 -> Gain7/1, Gain8/1
  Product/1 -> Gain5/1
  Constant/1 -> Product/1
  1-D Lookup Table/1 -> Add5/1
  Add5/1 -> Saturation4/1
  bra_pre_l/1 -> Add5/2
  Add4/1 -> [trq_dem_lf1]
  trq_dem_lf/1 -> Add4/2
  Gain4/1 -> Add4/1
  Add3/1 -> [trq_dem_lr1]
  trq_dem_lr/1 -> Add3/2
  Add2/1 -> Gain9/1
  s_act_lr/1 -> Sum/2
  Gain3/1 -> Difference/1
  Gain2/1 -> Discrete-Time Integrator/1
  Gain1/1 -> Add2/1
  Sum/1 -> Gain1/1, Gain3/1, Gain2/1
  s_opt_zhuan/1 -> Sum/1
  mot_drive/1 -> Mux/3
  mot_mode/1 -> Mux/2
  [trq_dem_lf1] -> Saturation/1
  mot_enable/1 -> Mux/1
  SpdSet_dem/1 -> Mux/5
  Mux/1 -> mot_lf/1
  TrqLim_dem/1 -> Mux/6
  HeartBeat/1(life) -> Mux/8, Memory/1
  Memory/1 -> HeartBeat/1(life_pre)
  SpdLim_dem/1 -> Mux/7
  mot_drive1/1 -> Mux2/3
  mot_mode2/1 -> Mux2/2
  trq_dem_rf/1 -> Saturation2/1
  mot_enable2/1 -> Mux2/1
  SpdSet_dem1/1 -> Mux2/5
  Mux2/1 -> mot_rf/1
  TrqLim_dem1/1 -> Mux2/6
  SpdLim_dem1/1 -> Mux2/7
  mot_drive2/1 -> Mux1/3
  mot_mode1/1 -> Mux1/2
  [trq_dem_lr1] -> Saturation1/1
  mot_enable1/1 -> Mux1/1
  SpdSet_dem2/1 -> Mux1/5
  Mux1/1 -> mot_lr/1
  TrqLim_dem2/1 -> Mux1/6
  HeartBeat1/1(life) -> Mux1/8, Memory1/1
  Memory1/1 -> HeartBeat1/1(life_pre)
  SpdLim_dem2/1 -> Mux1/7
  mot_drive3/1 -> Mux3/3
  mot_mode3/1 -> Mux3/2
  trq_dem_rr/1 -> Saturation3/1
  mot_enable3/1 -> Mux3/1
  SpdSet_dem3/1 -> Mux3/5
  Mux3/1 -> mot_rr/1
  TrqLim_dem3/1 -> Mux3/6
  SpdLim_dem3/1 -> Mux3/7
  Gain9/1 -> Add3/1, Gain4/1

== system analyze/MainControl/mode_control/backward/backward/Drive/驱动防滑控制TCS/转向TCS/右转/无滑转 ==
  trq_dem_lf : Inport
  trq_dem_lr : Inport  Port=2
  trq_dem_rf : Inport  Port=3
  trq_dem_rr : Inport  Port=4
  bra_pre_l : Inport  Port=5
  bra_pre_r : Inport  Port=6
  brake_dem : Inport  Port=7
  Action Port : ActionPort  ActionType=case
  1-D Lookup Table : Lookup_n-D  NumberOfTableDimensions=1  BreakpointsForDimension1=brakeTrq_dem_data  Table=brakepre_dem_data  InternalRulePriority=Speed  RndMeth=Simplest  InputSameDT=on
  1-D Lookup Table2 : Lookup_n-D  NumberOfTableDimensions=1  BreakpointsForDimension1=brakeTrq_dem_data  Table=brakepre_dem_data  InternalRulePriority=Speed  RndMeth=Simplest  InputSameDT=on
  Add2 : Sum
  Add3 : Sum
  Constant : Constant  Value=bratrq_max
  Gain1 : Gain  Gain=1/2
  Gain2 : Gain  Gain=1/100
  Gain3 : Gain  Gain=1/2
  Gain4 : Gain  Gain=1/2
  HeartBeat : MATLAB Function  TreatAsAtomicUnit=on
  HeartBeat1 : MATLAB Function  TreatAsAtomicUnit=on
  Memory : Memory  InheritSampleTime=on
  Memory1 : Memory  InheritSampleTime=on
  Mux : Mux  Inputs=8
  Mux1 : Mux  Inputs=8
  Mux2 : Mux  Inputs=7
  Mux3 : Mux  Inputs=7
  Product : Product
  Saturation{,1..3} (4 alike) : Saturate  UpperLimit=trqmax  LowerLimit=-trqmax
  Saturation4 : Saturate  UpperLimit=premax  LowerLimit=0
  Saturation5 : Saturate  UpperLimit=premax  LowerLimit=0
  SpdLim_dem{,1..3} (4 alike) : Constant  Value=spdmax
  SpdSet_dem{,1..3} (4 alike) : Constant
  TrqLim_dem{,1..3} (4 alike) : Constant
  mot_drive : Constant  Value=2
  mot_drive1 : Constant
  mot_drive2 : Constant  Value=2
  mot_drive3 : Constant
  mot_enable{,1..3} (4 alike) : Constant  Value=2
  mot_mode{,1..3} (4 alike) : Constant
  mot_lf : Outport
  mot_lr : Outport  Port=2
  mot_rf : Outport  Port=3
  mot_rr : Outport  Port=4
  bra_pre_l1 : Outport  Port=5
  bra_pre_r1 : Outport  Port=6
  wires:
  Saturation5/1 -> bra_pre_r1/1
  Saturation4/1 -> bra_pre_l1/1
  Saturation3/1 -> Mux3/4
  Saturation2/1 -> Mux2/4
  Saturation1/1 -> Mux1/4
  Saturation/1 -> Mux/4
  brake_dem/1 -> Gain2/1
  Add3/1 -> Saturation5/1
  bra_pre_r/1 -> Add3/2
  1-D Lookup Table2/1 -> Add3/1
  Gain4/1 -> 1-D Lookup Table2/1
  Gain3/1 -> 1-D Lookup Table/1
  Gain2/1 -> Product/2
  Gain1/1 -> Gain3/1, Gain4/1
  Product/1 -> Gain1/1
  Constant/1 -> Product/1
  1-D Lookup Table/1 -> Add2/1
  Add2/1 -> Saturation4/1
  bra_pre_l/1 -> Add2/2
  mot_drive/1 -> Mux/3
  mot_mode/1 -> Mux/2
  trq_dem_lf/1 -> Saturation/1
  mot_enable/1 -> Mux/1
  SpdSet_dem/1 -> Mux/5
  Mux/1 -> mot_lf/1
  TrqLim_dem/1 -> Mux/6
  HeartBeat/1(life) -> Mux/8, Memory/1
  Memory/1 -> HeartBeat/1(life_pre)
  SpdLim_dem/1 -> Mux/7
  mot_drive1/1 -> Mux2/3
  mot_mode2/1 -> Mux2/2
  trq_dem_rf/1 -> Saturation2/1
  mot_enable2/1 -> Mux2/1
  SpdSet_dem1/1 -> Mux2/5
  Mux2/1 -> mot_rf/1
  TrqLim_dem1/1 -> Mux2/6
  SpdLim_dem1/1 -> Mux2/7
  mot_drive2/1 -> Mux1/3
  mot_mode1/1 -> Mux1/2
  trq_dem_lr/1 -> Saturation1/1
  mot_enable1/1 -> Mux1/1
  SpdSet_dem2/1 -> Mux1/5
  Mux1/1 -> mot_lr/1
  TrqLim_dem2/1 -> Mux1/6
  HeartBeat1/1(life) -> Mux1/8, Memory1/1
  Memory1/1 -> HeartBeat1/1(life_pre)
  SpdLim_dem2/1 -> Mux1/7
  mot_drive3/1 -> Mux3/3
  mot_mode3/1 -> Mux3/2
  trq_dem_rr/1 -> Saturation3/1
  mot_enable3/1 -> Mux3/1
  SpdSet_dem3/1 -> Mux3/5
  Mux3/1 -> mot_rr/1
  TrqLim_dem3/1 -> Mux3/6
  SpdLim_dem3/1 -> Mux3/7

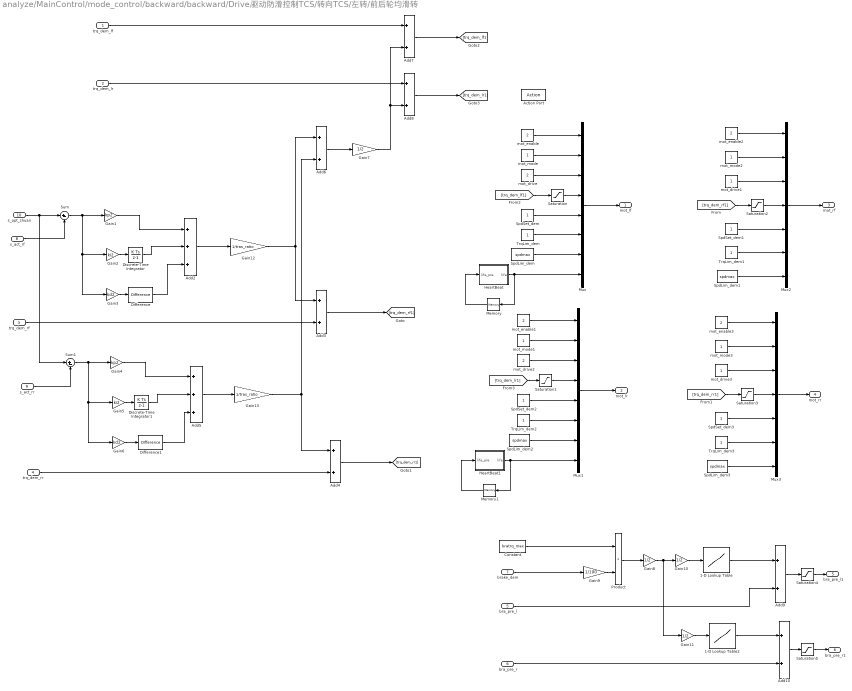
== system analyze/MainControl/mode_control/backward/backward/Drive/驱动防滑控制TCS/转向TCS/左转/前后轮均滑转 ==
  trq_dem_lf : Inport
  trq_dem_lr : Inport  Port=2
  trq_dem_rf : Inport  Port=3
  trq_dem_rr : Inport  Port=4
  bra_pre_l : Inport  Port=5
  bra_pre_r : Inport  Port=6
  brake_dem : Inport  Port=7
  s_act_rf : Inport  Port=8
  s_act_rr : Inport  Port=9
  s_opt_zhuan : Inport  Port=10
  Action Port : ActionPort  ActionType=case
  1-D Lookup Table : Lookup_n-D  NumberOfTableDimensions=1  BreakpointsForDimension1=brakeTrq_dem_data  Table=brakepre_dem_data  InternalRulePriority=Speed  RndMeth=Simplest  InputSameDT=on
  1-D Lookup Table2 : Lookup_n-D  NumberOfTableDimensions=1  BreakpointsForDimension1=brakeTrq_dem_data  Table=brakepre_dem_data  InternalRulePriority=Speed  RndMeth=Simplest  InputSameDT=on
  Add{3..4,6..10} (7 alike) : Sum
  Add2 : Sum  Inputs=+++
  Add5 : Sum  Inputs=+++
  Constant : Constant  Value=bratrq_max
  Difference : simulink/Discrete/Difference  ICPrevInput=0.0  InputProcessing=Inherited  OutMin=[]  OutMax=[]  OutDataType=fixdt(1, 16)  OutScaling=2^-10  DoSatur=off
  Difference1 : simulink/Discrete/Difference  ICPrevInput=0.0  InputProcessing=Inherited  OutMin=[]  OutMax=[]  OutDataType=fixdt(1, 16)  OutScaling=2^-10  DoSatur=off
  Discrete-Time Integrator : DiscreteIntegrator  SampleTime=-1  ICPrevOutput=DiscIntNeverNeededParam  ICPrevScaledInput=DiscIntNeverNeededParam
  Discrete-Time Integrator1 : DiscreteIntegrator  SampleTime=-1  ICPrevOutput=DiscIntNeverNeededParam  ICPrevScaledInput=DiscIntNeverNeededParam
  Gain1 : Gain  Gain=kp2
  Gain{7..8,10..11} (4 alike) : Gain  Gain=1/2
  Gain12 : Gain  Gain=1/tras_ratio
  Gain13 : Gain  Gain=1/tras_ratio
  Gain2 : Gain  Gain=ki2
  Gain3 : Gain  Gain=kd2
  Gain4 : Gain  Gain=kp2
  Gain5 : Gain  Gain=ki2
  Gain6 : Gain  Gain=kd2
  Gain9 : Gain  Gain=1/100
  HeartBeat : MATLAB Function  TreatAsAtomicUnit=on
  HeartBeat1 : MATLAB Function  TreatAsAtomicUnit=on
  Memory : Memory  InheritSampleTime=on
  Memory1 : Memory  InheritSampleTime=on
  Mux : Mux  Inputs=8
  Mux1 : Mux  Inputs=8
  Mux2 : Mux  Inputs=7
  Mux3 : Mux  Inputs=7
  Product : Product
  Saturation{,1..3} (4 alike) : Saturate  UpperLimit=trqmax  LowerLimit=-trqmax
  Saturation4 : Saturate  UpperLimit=premax  LowerLimit=0
  Saturation5 : Saturate  UpperLimit=premax  LowerLimit=0
  SpdLim_dem{,1..3} (4 alike) : Constant  Value=spdmax
  SpdSet_dem{,1..3} (4 alike) : Constant
  Sum : Sum  Inputs=|+-
  Sum1 : Sum  Inputs=|+-
  TrqLim_dem{,1..3} (4 alike) : Constant
  mot_drive : Constant  Value=2
  mot_drive1 : Constant
  mot_drive2 : Constant  Value=2
  mot_drive3 : Constant
  mot_enable{,1..3} (4 alike) : Constant  Value=2
  mot_mode{,1..3} (4 alike) : Constant
  mot_lf : Outport
  mot_lr : Outport  Port=2
  mot_rf : Outport  Port=3
  mot_rr : Outport  Port=4
  bra_pre_l1 : Outport  Port=5
  bra_pre_r1 : Outport  Port=6
  wires:
  Saturation5/1 -> bra_pre_r1/1
  Saturation4/1 -> bra_pre_l1/1
  Saturation3/1 -> Mux3/4
  Saturation2/1 -> Mux2/4
  Saturation1/1 -> Mux1/4
  Saturation/1 -> Mux/4
  Difference1/1 -> Add5/3
  Discrete-Time Integrator1/1 -> Add5/2
  Difference/1 -> Add2/3
  Discrete-Time Integrator/1 -> Add2/2
  brake_dem/1 -> Gain9/1
  Add10/1 -> Saturation5/1
  bra_pre_r/1 -> Add10/2
  1-D Lookup Table2/1 -> Add10/1
  Gain11/1 -> 1-D Lookup Table2/1
  Gain10/1 -> 1-D Lookup Table/1
  Gain9/1 -> Product/2
  Gain8/1 -> Gain10/1, Gain11/1
  Product/1 -> Gain8/1
  Constant/1 -> Product/1
  1-D Lookup Table/1 -> Add9/1
  Add9/1 -> Saturation4/1
  bra_pre_l/1 -> Add9/2
  Add8/1 -> [trq_dem_lr1]
  trq_dem_lr/1 -> Add8/1
  Add7/1 -> [trq_dem_lf1]
  Gain7/1 -> Add7/2, Add8/2
  trq_dem_lf/1 -> Add7/1
  Add6/1 -> Gain7/1
  trq_dem_rr/1 -> Add4/2
  Add5/1 -> Gain13/1
  s_act_rr/1 -> Sum1/2
  Gain6/1 -> Difference1/1
  Gain5/1 -> Discrete-Time Integrator1/1
  Gain4/1 -> Add5/1
  Sum1/1 -> Gain4/1, Gain6/1, Gain5/1
  Add4/1 -> [trq_dem_rr1]
  Add3/1 -> [trq_dem_rf1]
  trq_dem_rf/1 -> Add3/2
  Add2/1 -> Gain12/1
  s_act_rf/1 -> Sum/2
  Gain3/1 -> Difference/1
  Gain2/1 -> Discrete-Time Integrator/1
  Gain1/1 -> Add2/1
  Sum/1 -> Gain1/1, Gain3/1, Gain2/1
  s_opt_zhuan/1 -> Sum/1, Sum1/1
  mot_drive/1 -> Mux/3
  mot_mode/1 -> Mux/2
  [trq_dem_lf1] -> Saturation/1
  mot_enable/1 -> Mux/1
  SpdSet_dem/1 -> Mux/5
  Mux/1 -> mot_lf/1
  TrqLim_dem/1 -> Mux/6
  HeartBeat/1(life) -> Mux/8, Memory/1
  Memory/1 -> HeartBeat/1(life_pre)
  SpdLim_dem/1 -> Mux/7
  mot_drive1/1 -> Mux2/3
  mot_mode2/1 -> Mux2/2
  [trq_dem_rf1] -> Saturation2/1
  mot_enable2/1 -> Mux2/1
  SpdSet_dem1/1 -> Mux2/5
  Mux2/1 -> mot_rf/1
  TrqLim_dem1/1 -> Mux2/6
  SpdLim_dem1/1 -> Mux2/7
  mot_drive2/1 -> Mux1/3
  mot_mode1/1 -> Mux1/2
  [trq_dem_lr1] -> Saturation1/1
  mot_enable1/1 -> Mux1/1
  SpdSet_dem2/1 -> Mux1/5
  Mux1/1 -> mot_lr/1
  TrqLim_dem2/1 -> Mux1/6
  HeartBeat1/1(life) -> Mux1/8, Memory1/1
  Memory1/1 -> HeartBeat1/1(life_pre)
  SpdLim_dem2/1 -> Mux1/7
  mot_drive3/1 -> Mux3/3
  mot_mode3/1 -> Mux3/2
  [trq_dem_rr1] -> Saturation3/1
  mot_enable3/1 -> Mux3/1
  SpdSet_dem3/1 -> Mux3/5
  Mux3/1 -> mot_rr/1
  TrqLim_dem3/1 -> Mux3/6
  SpdLim_dem3/1 -> Mux3/7
  Gain12/1 -> Add6/1, Add3/1
  Gain13/1 -> Add6/2, Add4/1

== system analyze/MainControl/mode_control/backward/backward/Drive/驱动防滑控制TCS/转向TCS/左转/前轮滑转 ==
  trq_dem_lf : Inport
  trq_dem_lr : Inport  Port=2
  trq_dem_rf : Inport  Port=3
  trq_dem_rr : Inport  Port=4
  bra_pre_l : Inport  Port=5
  bra_pre_r : Inport  Port=6
  brake_dem : Inport  Port=7
  s_act_rf : Inport  Port=8
  s_opt_zhuan : Inport  Port=9
  Action Port : ActionPort  ActionType=case
  1-D Lookup Table : Lookup_n-D  NumberOfTableDimensions=1  BreakpointsForDimension1=brakeTrq_dem_data  Table=brakepre_dem_data  InternalRulePriority=Speed  RndMeth=Simplest  InputSameDT=on
  1-D Lookup Table2 : Lookup_n-D  NumberOfTableDimensions=1  BreakpointsForDimension1=brakeTrq_dem_data  Table=brakepre_dem_data  InternalRulePriority=Speed  RndMeth=Simplest  InputSameDT=on
  Add2 : Sum  Inputs=+++
  Add{3..6} (4 alike) : Sum
  Constant : Constant  Value=bratrq_max
  Difference : simulink/Discrete/Difference  ICPrevInput=0.0  InputProcessing=Inherited  OutMin=[]  OutMax=[]  OutDataType=fixdt(1, 16)  OutScaling=2^-10  DoSatur=off
  Discrete-Time Integrator : DiscreteIntegrator  SampleTime=-1  ICPrevOutput=DiscIntNeverNeededParam  ICPrevScaledInput=DiscIntNeverNeededParam
  Gain1 : Gain  Gain=kp2
  Gain2 : Gain  Gain=ki2
  Gain3 : Gain  Gain=kd2
  Gain4 : Gain  Gain=-1
  Gain5 : Gain  Gain=1/2
  Gain6 : Gain  Gain=1/100
  Gain7 : Gain  Gain=1/2
  Gain8 : Gain  Gain=1/2
  Gain9 : Gain  Gain=1/tras_ratio
  HeartBeat : MATLAB Function  TreatAsAtomicUnit=on
  HeartBeat1 : MATLAB Function  TreatAsAtomicUnit=on
  Memory : Memory  InheritSampleTime=on
  Memory1 : Memory  InheritSampleTime=on
  Mux : Mux  Inputs=8
  Mux1 : Mux  Inputs=8
  Mux2 : Mux  Inputs=7
  Mux3 : Mux  Inputs=7
  Product : Product
  Saturation{,1..3} (4 alike) : Saturate  UpperLimit=trqmax  LowerLimit=-trqmax
  Saturation4 : Saturate  UpperLimit=premax  LowerLimit=0
  Saturation5 : Saturate  UpperLimit=premax  LowerLimit=0
  SpdLim_dem{,1..3} (4 alike) : Constant  Value=spdmax
  SpdSet_dem{,1..3} (4 alike) : Constant
  Sum : Sum  Inputs=|+-
  TrqLim_dem{,1..3} (4 alike) : Constant
  mot_drive : Constant  Value=2
  mot_drive1 : Constant
  mot_drive2 : Constant  Value=2
  mot_drive3 : Constant
  mot_enable{,1..3} (4 alike) : Constant  Value=2
  mot_mode{,1..3} (4 alike) : Constant
  mot_lf : Outport
  mot_lr : Outport  Port=2
  mot_rf : Outport  Port=3
  mot_rr : Outport  Port=4
  bra_pre_l1 : Outport  Port=5
  bra_pre_r1 : Outport  Port=6
  wires:
  Saturation5/1 -> bra_pre_r1/1
  Saturation4/1 -> bra_pre_l1/1
  Saturation3/1 -> Mux3/4
  Saturation2/1 -> Mux2/4
  Saturation1/1 -> Mux1/4
  Saturation/1 -> Mux/4
  Difference/1 -> Add2/3
  Discrete-Time Integrator/1 -> Add2/2
  brake_dem/1 -> Gain6/1
  Add6/1 -> Saturation5/1
  bra_pre_r/1 -> Add6/2
  1-D Lookup Table2/1 -> Add6/1
  Gain8/1 -> 1-D Lookup Table2/1
  Gain7/1 -> 1-D Lookup Table/1
  Gain6/1 -> Product/2
  Gain5/1 -> Gain7/1, Gain8/1
  Product/1 -> Gain5/1
  Constant/1 -> Product/1
  1-D Lookup Table/1 -> Add5/1
  Add5/1 -> Saturation4/1
  bra_pre_l/1 -> Add5/2
  Add4/1 -> [trq_dem_rr1]
  trq_dem_rr/1 -> Add4/2
  Gain4/1 -> Add4/1
  Add3/1 -> [trq_dem_rf1]
  trq_dem_rf/1 -> Add3/2
  Add2/1 -> Gain9/1
  s_act_rf/1 -> Sum/2
  Gain3/1 -> Difference/1
  Gain2/1 -> Discrete-Time Integrator/1
  Gain1/1 -> Add2/1
  Sum/1 -> Gain1/1, Gain3/1, Gain2/1
  s_opt_zhuan/1 -> Sum/1
  mot_drive/1 -> Mux/3
  mot_mode/1 -> Mux/2
  trq_dem_lf/1 -> Saturation/1
  mot_enable/1 -> Mux/1
  SpdSet_dem/1 -> Mux/5
  Mux/1 -> mot_lf/1
  TrqLim_dem/1 -> Mux/6
  HeartBeat/1(life) -> Mux/8, Memory/1
  Memory/1 -> HeartBeat/1(life_pre)
  SpdLim_dem/1 -> Mux/7
  mot_drive1/1 -> Mux2/3
  mot_mode2/1 -> Mux2/2
  [trq_dem_rf1] -> Saturation2/1
  mot_enable2/1 -> Mux2/1
  SpdSet_dem1/1 -> Mux2/5
  Mux2/1 -> mot_rf/1
  TrqLim_dem1/1 -> Mux2/6
  SpdLim_dem1/1 -> Mux2/7
  mot_drive2/1 -> Mux1/3
  mot_mode1/1 -> Mux1/2
  trq_dem_lr/1 -> Saturation1/1
  mot_enable1/1 -> Mux1/1
  SpdSet_dem2/1 -> Mux1/5
  Mux1/1 -> mot_lr/1
  TrqLim_dem2/1 -> Mux1/6
  HeartBeat1/1(life) -> Mux1/8, Memory1/1
  Memory1/1 -> HeartBeat1/1(life_pre)
  SpdLim_dem2/1 -> Mux1/7
  mot_drive3/1 -> Mux3/3
  mot_mode3/1 -> Mux3/2
  [trq_dem_rr1] -> Saturation3/1
  mot_enable3/1 -> Mux3/1
  SpdSet_dem3/1 -> Mux3/5
  Mux3/1 -> mot_rr/1
  TrqLim_dem3/1 -> Mux3/6
  SpdLim_dem3/1 -> Mux3/7
  Gain9/1 -> Add3/1, Gain4/1
